simulink model "PID_controller"  (R2020a)
settings: Solver=VariableStepAuto  StartTime=0.0  StopTime=50  RelTol=1e-3
settings Model: Creator=Administrator  LastModifiedBy=Administrator

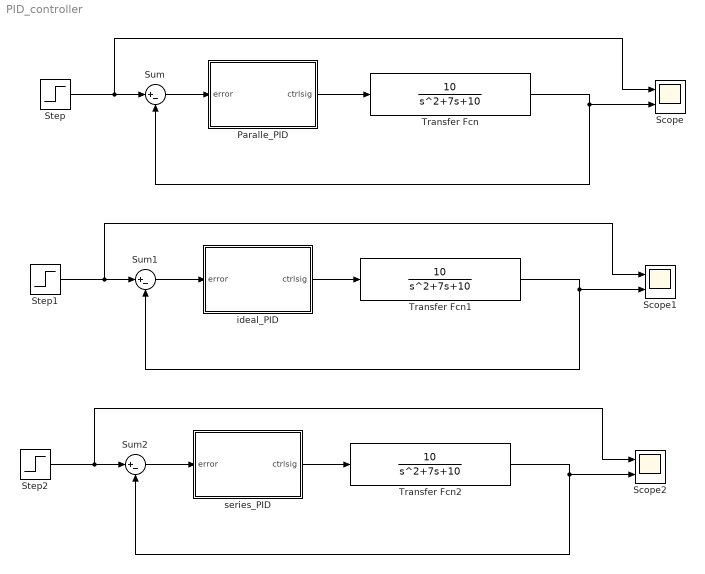
== system PID_controller ==
  Paralle_PID : Subsystem
  Scope : Scope  NumInputPorts=2
  Scope1 : Scope  NumInputPorts=2
  Scope2 : Scope  NumInputPorts=2
  Step : Step  SampleTime=0
  Step1 : Step  SampleTime=0
  Step2 : Step  SampleTime=0
  Sum : Sum  Inputs=|+-
  Sum1 : Sum  Inputs=|+-
  Sum2 : Sum  Inputs=|+-
  Transfer Fcn : TransferFcn  Numerator=[10]  Denominator=[1 7 10]
  Transfer Fcn1 : TransferFcn  Numerator=[10]  Denominator=[1 7 10]
  Transfer Fcn2 : TransferFcn  Numerator=[10]  Denominator=[1 7 10]
  ideal_PID : Subsystem
  series_PID : Subsystem
  wires:
  Paralle_PID/1(ctrlsig) -> Transfer Fcn/1
  Step/1 -> Scope/1, Sum/1
  Sum/1 -> Paralle_PID/1(error)
  Transfer Fcn/1 -> Scope/2, Sum/2
  Transfer Fcn1/1 -> Sum1/2, Scope1/2
  Sum1/1 -> ideal_PID/1(error)
  Step1/1 -> Sum1/1, Scope1/1
  ideal_PID/1(ctrlsig) -> Transfer Fcn1/1
  series_PID/1(ctrlsig) -> Transfer Fcn2/1
  Step2/1 -> Scope2/1, Sum2/1
  Sum2/1 -> series_PID/1(error)
  Transfer Fcn2/1 -> Scope2/2, Sum2/2

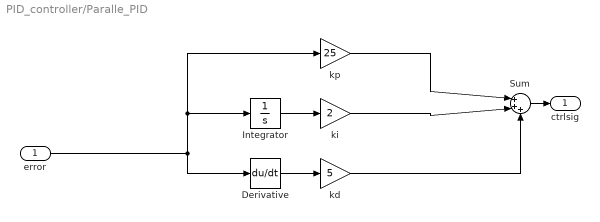
== system PID_controller/Paralle_PID ==
  error : Inport
  Derivative : Derivative
  Integrator : Integrator
  Sum : Sum  Inputs=|+++
  kd : Gain  Gain=5
  ki : Gain  Gain=2
  kp : Gain  Gain=25
  ctrlsig : Outport
  wires:
  error/1 -> Derivative/1, Integrator/1, kp/1
  ki/1 -> Sum/2
  Integrator/1 -> ki/1
  Sum/1 -> ctrlsig/1
  Derivative/1 -> kd/1
  kd/1 -> Sum/3
  kp/1 -> Sum/1

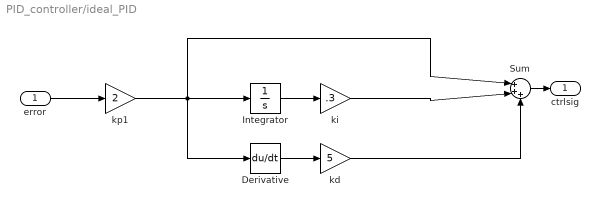
== system PID_controller/ideal_PID ==
  error : Inport
  Derivative : Derivative
  Integrator : Integrator
  Sum : Sum  Inputs=|+++
  kd : Gain  Gain=5
  ki : Gain  Gain=.3
  kp1 : Gain  Gain=2
  ctrlsig : Outport
  wires:
  kp1/1 -> Derivative/1, Sum/1, Integrator/1
  kd/1 -> Sum/3
  Derivative/1 -> kd/1
  Sum/1 -> ctrlsig/1
  Integrator/1 -> ki/1
  ki/1 -> Sum/2
  error/1 -> kp1/1

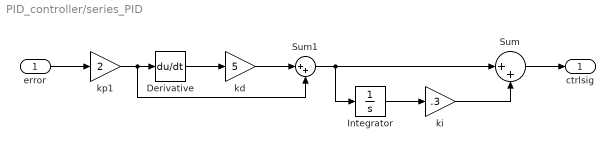
== system PID_controller/series_PID ==
  error : Inport
  Derivative : Derivative
  Integrator : Integrator
  Sum : Sum  Inputs=|++
  Sum1 : Sum  Inputs=|++
  kd : Gain  Gain=5
  ki : Gain  Gain=.3
  kp1 : Gain  Gain=2
  ctrlsig : Outport
  wires:
  error/1 -> kp1/1
  ki/1 -> Sum/2
  Integrator/1 -> ki/1
  Sum/1 -> ctrlsig/1
  Derivative/1 -> kd/1
  kd/1 -> Sum1/1
  Sum1/1 -> Integrator/1, Sum/1
  kp1/1 -> Derivative/1, Sum1/2
